simulink model "generic"  (R2022b)
settings: Solver=ode45  StartTime=0.0  StopTime=inf  RelTol=1e-3  EnableMultiTasking=on
values from neighbouring files (symbols this model uses):
  A = cell2mat(A_cell)    [MPCController1.m]    (also in MPC_Fmincon.m)
  B = cell2mat(B_cell)    [MPCController1.m]    (also in MPC_Fmincon.m)
  brake_select = ones(length(speed), length(steering_angle))    [TwoDLook_uptable.m]
  curvature = 0.000:0.001:1    [TwoDLook_uptable.m]
  m = 1600    [MPCController1.m]    (also in MPCController2.m; MPC_Fmincon.m)
  speed = 0:0.1:100    [TwoDLook_uptable.m]
undefined symbols (not defined in the file or in its folder): Amplifier, DiscIntNeverNeededParam, K_d_yawrate, K_dsteering, k_speed, k_stanley, kd, ki, kp, path_curvature
libraries: CarMaker4SL x97, simulink x6, cstblocks x6, simulink_extras x4, autolibshared x1, mpcadaslib x1
(part 4 of 6)

== system generic/CarMaker/VehicleControl/CreateBus VhclCtrl1/Stanley steering & speed//Brake controller/Stanley_controller_with_thottle_and_brake_commands/Stanley steering + PID speed controller/Smoothing ==
  Signal_In : Inport
  Add : Sum  Inputs=++++
  Delay : Delay  InitialCondition=0.1
  Delay1 : Delay  DelayLength=4  InitialCondition=0.1
  Delay2 : Delay  DelayLength=5  InitialCondition=0.1
  Gain : Gain  Gain=0.35
  Gain1 : Gain  Gain=0.25
  Gain2 : Gain  Gain=0.25
  Gain3 : Gain  Gain=0.15
  Signal_Out : Outport  VectorParamsAs1DForOutWhenUnconnected=off
  wires:
  Gain1/1 -> Add/2
  Signal_In/1 -> Gain/1
  Delay/1 -> Gain1/1
  Gain/1 -> Add/1
  Delay1/1 -> Gain2/1
  Add/1 -> Delay2/1, Delay1/1, Delay/1, Signal_Out/1
  Gain2/1 -> Add/3
  Delay2/1 -> Gain3/1
  Gain3/1 -> Add/4

== system generic/CarMaker/VehicleControl/CreateBus VhclCtrl1/Stanley steering & speed//Brake controller/Stanley_controller_with_thottle_and_brake_commands/Stanley steering + PID speed controller/Speed_controller ==
  path : Inport
  speed_act : Inport  Port=2
  velocity_x : Inport  Port=3
  velocity_y : Inport  Port=4
  desired_speed : Inport  Port=5
  steering : Inport  Port=6
  Brake Saturation : Saturate  UpperLimit=1  LowerLimit=0
  Constant1 : Constant  Value=kd
  Constant2 : Constant  Value=ki
  Constant3 : Constant  Value=kp
  Path_curvature : Constant  Value=path_curvature
  Scaling factor : Gain  Gain=1/1000
  Scalling factor : Gain  Gain=1/1000
  Throttle Saturation : Saturate  UpperLimit=1  LowerLimit=-1
  advancedPID_speed_and_brake_control : MATLAB Function  TreatAsAtomicUnit=on
  calculate_path_curvature : MATLAB Function  TreatAsAtomicUnit=on
  Throttle : Outport
  Brake_command : Outport  Port=2
  path_curvature : Outport  Port=3
  min_safe_speed : Outport  Port=4
  wires:
  advancedPID_speed_and_brake_control/1(throttle) -> Scaling factor/1  "throttle"
  path/1 -> calculate_path_curvature/1(path)
  speed_act/1 -> advancedPID_speed_and_brake_control/3(speed_act)
  calculate_path_curvature/2(min_safe_speed) -> min_safe_speed/1, advancedPID_speed_and_brake_control/2(min_s_speed)  "min_s_speed"
  velocity_y/1 -> calculate_path_curvature/2(velocity_y)
  velocity_x/1 -> calculate_path_curvature/3(velocity_x)
  steering/1 -> calculate_path_curvature/4(steering_angel)
  calculate_path_curvature/1(path_curvature) -> path_curvature/1
  Constant3/1 -> advancedPID_speed_and_brake_control/7(Kp_speed)
  Path_curvature/1 -> advancedPID_speed_and_brake_control/1(path_curv)
  desired_speed/1 -> advancedPID_speed_and_brake_control/4(desired_speed)
  Constant2/1 -> advancedPID_speed_and_brake_control/6(Ki_speed)
  Constant1/1 -> advancedPID_speed_and_brake_control/5(Kd_speed)
  advancedPID_speed_and_brake_control/2(brake_cmd) -> Scalling factor/1  "Brake cmd"
  Scaling factor/1 -> Throttle Saturation/1
  Throttle Saturation/1 -> Throttle/1  "Throttle_command"
  Scalling factor/1 -> Brake Saturation/1
  Brake Saturation/1 -> Brake_command/1  "Brake_command"

== system generic/CarMaker/VehicleControl/CreateBus VhclCtrl1/Stanley steering & speed//Brake controller/Stanley_controller_with_thottle_and_brake_commands/Stanley steering + PID speed controller/Subsystem1 ==
  desired_speed : Inport
  curvature : Inport  Port=2
  min_safe_speed : Inport  Port=3
  2-D Lookup Table : Lookup_n-D  BreakpointsForDimension1=speed  BreakpointsForDimension2=curvature  Table=brake_select  InternalRulePriority=Speed  RndMeth=Simplest
      settings: InputPortMap=u0,u1
  Divide : Product  Inputs=*/
  MATLAB Function : MATLAB Function  Commented=on  TreatAsAtomicUnit=on
  Read CM Dict : CarMaker4SL/Read CM Dict  xname=Sensor.Road.VehSensor_0.Path.CurveXY  xsync=off  xstime=Continuous
  Scope2 : Scope
  Target_speed : Outport
  curv : Outport  Port=2
  speed : Outport  Port=3
  wires:
  Divide/1 -> speed/1, Target_speed/1, Scope2/1
  2-D Lookup Table/1 -> Divide/2
  desired_speed/1 -> 2-D Lookup Table/1, Divide/1
  min_safe_speed/1 -> MATLAB Function/2(min_safe_speed)
  curvature/1 -> MATLAB Function/1(u)
  Read CM Dict/1 -> curv/1, 2-D Lookup Table/2

== system generic/CarMaker/VehicleControl/CreateBus VhclCtrl1/Stanley steering & speed//Brake controller/Road sensor set & path planning/Road sensor set & path planning/A* star path planning/Signal_smoothing ==
  Signal_In : Inport
  Smoothing1 : Subsystem
  Smoothing2 : Subsystem
  Smoothing4 : Subsystem
  smoothed_width : Outport
  wires:
  Signal_In/1 -> Smoothing1/1(Signal_In)
  Smoothing1/1(Signal_Out) -> Smoothing2/1(Signal_In)  "steering_signal"
  Smoothing2/1(Signal_Out) -> Smoothing4/1(Signal_In)  "steering_signal"
  Smoothing4/1(Signal_Out) -> smoothed_width/1  "smoothed_width"

== system generic/CarMaker/VehicleControl/CreateBus VhclCtrl1/Stanley steering & speed//Brake controller/Road sensor set & path planning/Road sensor set & path planning/A* star path planning/Smoothing3 ==
  Signal_In : Inport
  Add : Sum  Inputs=++++
  Delay : Delay  InitialCondition=0.1
  Delay1 : Delay  DelayLength=4  InitialCondition=0.1
  Delay2 : Delay  DelayLength=5  InitialCondition=0.1
  Gain : Gain  Gain=0.35
  Gain1 : Gain  Gain=0.25
  Gain2 : Gain  Gain=0.25
  Gain3 : Gain  Gain=0.15
  Signal_Out : Outport  VectorParamsAs1DForOutWhenUnconnected=off
  wires:
  Gain3/1 -> Add/4
  Delay2/1 -> Gain3/1
  Gain2/1 -> Add/3
  Add/1 -> Signal_Out/1, Delay/1, Delay1/1, Delay2/1
  Delay1/1 -> Gain2/1
  Gain/1 -> Add/1
  Delay/1 -> Gain1/1
  Signal_In/1 -> Gain/1
  Gain1/1 -> Add/2

== system generic/CarMaker/VehicleControl/CreateBus VhclCtrl1/Stanley steering & speed//Brake controller/Road sensor set & path planning/Road sensor set & path planning/Be'zeir path planning/Signal_smoothing ==
  Signal_In : Inport
  Smoothing1 : Subsystem
  Smoothing2 : Subsystem
  Smoothing4 : Subsystem
  smoothed_width : Outport
  wires:
  Smoothing4/1(Signal_Out) -> smoothed_width/1  "smoothed_width"
  Smoothing2/1(Signal_Out) -> Smoothing4/1(Signal_In)  "steering_signal"
  Smoothing1/1(Signal_Out) -> Smoothing2/1(Signal_In)  "steering_signal"
  Signal_In/1 -> Smoothing1/1(Signal_In)

== system generic/CarMaker/VehicleControl/CreateBus VhclCtrl1/Stanley steering & speed//Brake controller/Road sensor set & path planning/Road sensor set & path planning/Be'zeir path planning/Smoothing3 ==
  Signal_In : Inport
  Add : Sum  Inputs=++++
  Delay : Delay  InitialCondition=0.1
  Delay1 : Delay  DelayLength=4  InitialCondition=0.1
  Delay2 : Delay  DelayLength=5  InitialCondition=0.1
  Gain : Gain  Gain=0.35
  Gain1 : Gain  Gain=0.25
  Gain2 : Gain  Gain=0.25
  Gain3 : Gain  Gain=0.15
  Signal_Out : Outport  VectorParamsAs1DForOutWhenUnconnected=off
  wires:
  Gain1/1 -> Add/2
  Signal_In/1 -> Gain/1
  Delay/1 -> Gain1/1
  Gain/1 -> Add/1
  Delay1/1 -> Gain2/1
  Add/1 -> Delay2/1, Delay1/1, Delay/1, Signal_Out/1
  Gain2/1 -> Add/3
  Delay2/1 -> Gain3/1
  Gain3/1 -> Add/4

== system generic/CarMaker/VehicleControl/CreateBus VhclCtrl1/Stanley steering & speed//Brake controller/Road sensor set & path planning/Road sensor set & path planning/Car_yaw_rate/ Path_expanding1 ==
  X-path : Inport
  Y_path : Inport  Port=2
  Delay10 : Delay  DelayLength=6
  Delay11 : Delay  DelayLength=8
  Delay37 : Delay
  Delay38 : Delay  DelayLength=4
  Delay4 : Delay
  Delay5 : Delay  DelayLength=6
  Delay6 : Delay  DelayLength=8
  Delay9 : Delay  DelayLength=4
  Mux1 : Mux  Inputs=5
  Mux2 : Mux  Inputs=5
  Reshape1 : Reshape  OutputDimensionality=Customize  OutputDimensions=[1,5]
  Reshape2 : Reshape  OutputDimensionality=Customize  OutputDimensions=[1,5]
  x_path : Outport
  y_path : Outport  Port=2
  wires:
  Mux2/1 -> Reshape2/1
  Reshape2/1 -> x_path/1
  Delay11/1 -> Mux1/5
  Delay10/1 -> Mux1/4
  Delay9/1 -> Mux1/3
  Delay4/1 -> Mux1/2
  Reshape1/1 -> y_path/1
  Mux1/1 -> Reshape1/1
  Delay38/1 -> Mux2/3
  Delay6/1 -> Mux2/5
  Delay37/1 -> Mux2/2
  Delay5/1 -> Mux2/4
  Y_path/1 -> Delay11/1, Delay10/1, Delay9/1, Delay4/1, Mux1/1
  X-path/1 -> Delay6/1, Delay5/1, Delay37/1, Delay38/1, Mux2/1

== system generic/CarMaker/VehicleControl/CreateBus VhclCtrl1/Stanley steering & speed//Brake controller/Road sensor set & path planning/Road sensor set & path planning/Dijkestra path planning/Signal_smoothing ==
  Signal_In : Inport
  Smoothing1 : Subsystem
  Smoothing2 : Subsystem
  Smoothing4 : Subsystem
  smoothed_width : Outport
  wires:
  Smoothing4/1(Signal_Out) -> smoothed_width/1  "smoothed_width"
  Smoothing2/1(Signal_Out) -> Smoothing4/1(Signal_In)  "steering_signal"
  Smoothing1/1(Signal_Out) -> Smoothing2/1(Signal_In)  "steering_signal"
  Signal_In/1 -> Smoothing1/1(Signal_In)

== system generic/CarMaker/VehicleControl/CreateBus VhclCtrl1/Stanley steering & speed//Brake controller/Road sensor set & path planning/Road sensor set & path planning/Dijkestra path planning/Smoothing3 ==
  Signal_In : Inport
  Add : Sum  Inputs=++++
  Delay : Delay  InitialCondition=0.1
  Delay1 : Delay  DelayLength=4  InitialCondition=0.1
  Delay2 : Delay  DelayLength=5  InitialCondition=0.1
  Gain : Gain  Gain=0.35
  Gain1 : Gain  Gain=0.25
  Gain2 : Gain  Gain=0.25
  Gain3 : Gain  Gain=0.15
  Signal_Out : Outport  VectorParamsAs1DForOutWhenUnconnected=off
  wires:
  Gain1/1 -> Add/2
  Signal_In/1 -> Gain/1
  Delay/1 -> Gain1/1
  Gain/1 -> Add/1
  Delay1/1 -> Gain2/1
  Add/1 -> Delay2/1, Delay1/1, Delay/1, Signal_Out/1
  Gain2/1 -> Add/3
  Delay2/1 -> Gain3/1
  Gain3/1 -> Add/4

== system generic/CarMaker/VehicleControl/CreateBus VhclCtrl1/Stanley steering & speed//Brake controller/Road sensor set & path planning/Road sensor set & path planning/Path_curvature/ Path_expanding ==
  X-path : Inport
  Y_path : Inport  Port=2
  Delay10 : Delay  DelayLength=6
  Delay11 : Delay  DelayLength=8
  Delay37 : Delay
  Delay38 : Delay  DelayLength=4
  Delay4 : Delay
  Delay5 : Delay  DelayLength=6
  Delay6 : Delay  DelayLength=8
  Delay9 : Delay  DelayLength=4
  Mux1 : Mux  Inputs=5
  Mux2 : Mux  Inputs=5
  Reshape1 : Reshape  OutputDimensionality=Customize  OutputDimensions=[1,5]
  Reshape2 : Reshape  OutputDimensionality=Customize  OutputDimensions=[1,5]
  x_path : Outport
  y_path : Outport  Port=2
  wires:
  X-path/1 -> Mux2/1, Delay38/1, Delay37/1, Delay5/1, Delay6/1
  Y_path/1 -> Mux1/1, Delay4/1, Delay9/1, Delay10/1, Delay11/1
  Delay5/1 -> Mux2/4
  Delay37/1 -> Mux2/2
  Delay6/1 -> Mux2/5
  Delay38/1 -> Mux2/3
  Mux1/1 -> Reshape1/1
  Reshape1/1 -> y_path/1
  Delay4/1 -> Mux1/2
  Delay9/1 -> Mux1/3
  Delay10/1 -> Mux1/4
  Delay11/1 -> Mux1/5
  Reshape2/1 -> x_path/1
  Mux2/1 -> Reshape2/1

== system generic/CarMaker/VehicleControl/CreateBus VhclCtrl1/Stanley steering & speed//Brake controller/Road sensor set & path planning/Road sensor set & path planning/Spline_path_planning/Signal_smoothing ==
  Signal_In : Inport
  Smoothing1 : Subsystem
  Smoothing2 : Subsystem
  Smoothing4 : Subsystem
  smoothed_width : Outport
  wires:
  Signal_In/1 -> Smoothing1/1(Signal_In)
  Smoothing1/1(Signal_Out) -> Smoothing2/1(Signal_In)  "steering_signal"
  Smoothing2/1(Signal_Out) -> Smoothing4/1(Signal_In)  "steering_signal"
  Smoothing4/1(Signal_Out) -> smoothed_width/1  "smoothed_width"

== system generic/CarMaker/VehicleControl/CreateBus VhclCtrl1/Stanley steering & speed//Brake controller/Road sensor set & path planning/Road sensor set & path planning/Spline_path_planning/Smoothing3 ==
  Signal_In : Inport
  Add : Sum  Inputs=++++
  Delay : Delay  InitialCondition=0.1
  Delay1 : Delay  DelayLength=4  InitialCondition=0.1
  Delay2 : Delay  DelayLength=5  InitialCondition=0.1
  Gain : Gain  Gain=0.35
  Gain1 : Gain  Gain=0.25
  Gain2 : Gain  Gain=0.25
  Gain3 : Gain  Gain=0.15
  Signal_Out : Outport  VectorParamsAs1DForOutWhenUnconnected=off
  wires:
  Gain3/1 -> Add/4
  Delay2/1 -> Gain3/1
  Gain2/1 -> Add/3
  Add/1 -> Signal_Out/1, Delay/1, Delay1/1, Delay2/1
  Delay1/1 -> Gain2/1
  Gain/1 -> Add/1
  Delay/1 -> Gain1/1
  Signal_In/1 -> Gain/1
  Gain1/1 -> Add/2

== system generic/CarMaker/VehicleControl/CreateBus VhclCtrl1/Stanley steering & speed//Brake controller/Road sensor set & path planning/Road sensor set & path planning/path_planning/Signal_smoothing ==
  Signal_In : Inport
  Smoothing1 : Subsystem
  Smoothing2 : Subsystem
  Smoothing4 : Subsystem
  smoothed_width : Outport
  wires:
  Smoothing4/1(Signal_Out) -> smoothed_width/1  "smoothed_width"
  Smoothing2/1(Signal_Out) -> Smoothing4/1(Signal_In)  "steering_signal"
  Smoothing1/1(Signal_Out) -> Smoothing2/1(Signal_In)  "steering_signal"
  Signal_In/1 -> Smoothing1/1(Signal_In)

== system generic/CarMaker/VehicleControl/CreateBus VhclCtrl1/Stanley steering & speed//Brake controller/Road sensor set & path planning/Road sensor set & path planning/path_planning/Smoothing3 ==
  Signal_In : Inport
  Add : Sum  Inputs=++++
  Delay : Delay  InitialCondition=0.1
  Delay1 : Delay  DelayLength=4  InitialCondition=0.1
  Delay2 : Delay  DelayLength=5  InitialCondition=0.1
  Gain : Gain  Gain=0.35
  Gain1 : Gain  Gain=0.25
  Gain2 : Gain  Gain=0.25
  Gain3 : Gain  Gain=0.15
  Signal_Out : Outport  VectorParamsAs1DForOutWhenUnconnected=off
  wires:
  Gain1/1 -> Add/2
  Signal_In/1 -> Gain/1
  Delay/1 -> Gain1/1
  Gain/1 -> Add/1
  Delay1/1 -> Gain2/1
  Add/1 -> Delay2/1, Delay1/1, Delay/1, Signal_Out/1
  Gain2/1 -> Add/3
  Delay2/1 -> Gain3/1
  Gain3/1 -> Add/4

== system generic/CarMaker/VehicleControl/CreateBus VhclCtrl1/Stanley steering & speed//Brake controller/Stanley_controller_vfin/Stanley_controller_vfin/Stanley_standfort controller/Crosstrack_steering ==
  speed : Inport
  Path.DevDist : Inport  Port=2
  Atan : Trigonometry  Operator=atan
  Divide : Product  Inputs=*/
  Gain : Gain  Gain=-1
  Product : Product
  Sum1 : Sum  Inputs=|++
  k_speed : Constant  Value=k_speed
  k_stanley : Constant  Value=k_stanley
  Cross_track_steering : Outport
  wires:
  Atan/1 -> Cross_track_steering/1
  Divide/1 -> Atan/1
  k_speed/1 -> Sum1/1
  speed/1 -> Sum1/2
  k_stanley/1 -> Product/2
  Sum1/1 -> Divide/2
  Product/1 -> Gain/1
  Gain/1 -> Divide/1
  Path.DevDist/1 -> Product/1

== system generic/CarMaker/VehicleControl/CreateBus VhclCtrl1/Stanley steering & speed//Brake controller/Stanley_controller_vfin/Stanley_controller_vfin/Stanley_standfort controller/Deviation_angle_calc ==
  Velocity : Inport
  Curvature : Inport  Port=2
  Car.YawRate : Inport  Port=3
  Amplifyer : Gain  Gain=Amplifier
  Amplifyer1 : Gain  Gain=10
  Amplifyer2 : Gain  Gain=16.56
  Constant : Constant  Value=2
  Discrete-Time Integrator : DiscreteIntegrator  SampleTime=-1  ICPrevOutput=DiscIntNeverNeededParam  ICPrevScaledInput=DiscIntNeverNeededParam
  Integrator : DiscreteIntegrator  SampleTime=-1  ICPrevOutput=DiscIntNeverNeededParam  ICPrevScaledInput=DiscIntNeverNeededParam
  Multiport Switch : MultiPortSwitch  Inputs=2  SaturateOnIntegerOverflow=off  InputSameDT=off
  Product : Product
  Read CM Dict : CarMaker4SL/Read CM Dict  xname=Sensor.Road.VehSensor_0.Path.DevAng  xsync=off  xstime=Continuous
  Scope : Scope  NumInputPorts=2
  Sum3 : Sum  Inputs=|+-
  Switch : Switch  Criteria=u2 > Threshold  SaturateOnIntegerOverflow=off  InputSameDT=off
  Dev_angle : Outport
  wires:
  Amplifyer1/1 -> Switch/3  "Dev_angle"
  Curvature/1 -> Product/1
  Car.YawRate/1 -> Discrete-Time Integrator/1
  Velocity/1 -> Product/2
  Product/1 -> Integrator/1
  Integrator/1 -> Sum3/1  "Dev_angle"
  Discrete-Time Integrator/1 -> Sum3/2
  Amplifyer2/1 -> Switch/1  "Dev_angle"
  Sum3/1 -> Amplifyer1/1, Switch/2, Amplifyer2/1  "heading_error"
  Switch/1 -> Scope/1, Multiport Switch/2  "Dev_angle"
  Amplifyer/1 -> Scope/2, Multiport Switch/3  "Dev_angle"
  Read CM Dict/1 -> Amplifyer/1
  Constant/1 -> Multiport Switch/1
  Multiport Switch/1 -> Dev_angle/1  "Dev_angle"

== system generic/CarMaker/VehicleControl/CreateBus VhclCtrl1/Stanley steering & speed//Brake controller/Stanley_controller_vfin/Stanley_controller_vfin/Stanley_standfort controller/Steady_state_yaw ==
  V : Inport
  Curvature : Inport  Port=2
  Car_Yaw_rate : Inport  Port=3
  Discrete-Time Integrator : DiscreteIntegrator  SampleTime=-1  ICPrevOutput=DiscIntNeverNeededParam  ICPrevScaledInput=DiscIntNeverNeededParam
  Steady_state_yaw : Subsystem
  Sum : Sum  Inputs=|-+
  Steady_state_yaw1 : Outport
  wires:
  V/1 -> Steady_state_yaw/1(V)
  Sum/1 -> Steady_state_yaw1/1  "Steady_state_yaw"
  Steady_state_yaw/1(Steady_state_yaw) -> Sum/1  "Steady_state_yaw"
  Discrete-Time Integrator/1 -> Sum/2
  Car_Yaw_rate/1 -> Discrete-Time Integrator/1
  Curvature/1 -> Steady_state_yaw/2(Curvature)

== system generic/CarMaker/VehicleControl/CreateBus VhclCtrl1/Stanley steering & speed//Brake controller/Stanley_controller_vfin/Stanley_controller_vfin/Stanley_standfort controller/Steering_correction_facotr ==
  Steering_i+1 : Inport
  Steering_i : Inport  Port=2
  K_dsteering : Constant  Value=K_dsteering
  Memory : Memory  LinearizeAsDelay=on
  Product2 : Product
  Sum2 : Sum  Inputs=|+-
  Factor_of_correction : Outport
  wires:
  K_dsteering/1 -> Product2/1
  Memory/1 -> Sum2/1
  Sum2/1 -> Product2/2
  Steering_i+1/1 -> Sum2/2
  Steering_i/1 -> Memory/1
  Product2/1 -> Factor_of_correction/1

== system generic/CarMaker/VehicleControl/CreateBus VhclCtrl1/Stanley steering & speed//Brake controller/Stanley_controller_vfin/Stanley_controller_vfin/Stanley_standfort controller/Yaw_rate_diff ==
  Velocity : Inport
  Curvature : Inport  Port=2
  Car_yaw_rate : Inport  Port=3
  K_d_yawrate : Constant  Value=K_d_yawrate
  Product : Product
  Product1 : Product
  Sum1 : Sum  Inputs=|+-
  Yaw_rate_factor : Outport
  wires:
  K_d_yawrate/1 -> Product1/1
  Car_yaw_rate/1 -> Sum1/2
  Velocity/1 -> Product/1
  Curvature/1 -> Product/2
  Sum1/1 -> Product1/2
  Product/1 -> Sum1/1
  Product1/1 -> Yaw_rate_factor/1

== system generic/CarMaker/VehicleControl/CreateBus VhclCtrl1/Stanley steering & speed//Brake controller/Road sensor set & path planning/Road sensor set & path planning/A* star path planning/Signal_smoothing/Smoothing1 ==
  Signal_In : Inport
  Add : Sum  Inputs=++++
  Delay : Delay  InitialCondition=0.1
  Delay1 : Delay  DelayLength=4  InitialCondition=0.1
  Delay2 : Delay  DelayLength=5  InitialCondition=0.1
  Gain : Gain  Gain=0.35
  Gain1 : Gain  Gain=0.25
  Gain2 : Gain  Gain=0.25
  Gain3 : Gain  Gain=0.15
  Signal_Out : Outport  VectorParamsAs1DForOutWhenUnconnected=off
  wires:
  Gain1/1 -> Add/2
  Signal_In/1 -> Gain/1
  Delay/1 -> Gain1/1
  Gain/1 -> Add/1
  Delay1/1 -> Gain2/1
  Add/1 -> Delay2/1, Delay1/1, Delay/1, Signal_Out/1
  Gain2/1 -> Add/3
  Delay2/1 -> Gain3/1
  Gain3/1 -> Add/4

== system generic/CarMaker/VehicleControl/CreateBus VhclCtrl1/Stanley steering & speed//Brake controller/Road sensor set & path planning/Road sensor set & path planning/A* star path planning/Signal_smoothing/Smoothing2 ==
  Signal_In : Inport
  Add : Sum  Inputs=++++
  Delay : Delay  InitialCondition=0.1
  Delay1 : Delay  DelayLength=4  InitialCondition=0.1
  Delay2 : Delay  DelayLength=5  InitialCondition=0.1
  Gain : Gain  Gain=0.35
  Gain1 : Gain  Gain=0.25
  Gain2 : Gain  Gain=0.25
  Gain3 : Gain  Gain=0.15
  Signal_Out : Outport  VectorParamsAs1DForOutWhenUnconnected=off
  wires:
  Gain3/1 -> Add/4
  Delay2/1 -> Gain3/1
  Gain2/1 -> Add/3
  Add/1 -> Signal_Out/1, Delay/1, Delay1/1, Delay2/1
  Delay1/1 -> Gain2/1
  Gain/1 -> Add/1
  Delay/1 -> Gain1/1
  Signal_In/1 -> Gain/1
  Gain1/1 -> Add/2

== system generic/CarMaker/VehicleControl/CreateBus VhclCtrl1/Stanley steering & speed//Brake controller/Road sensor set & path planning/Road sensor set & path planning/A* star path planning/Signal_smoothing/Smoothing4 ==
  Signal_In : Inport
  Add : Sum  Inputs=++++
  Delay : Delay  InitialCondition=0.1
  Delay1 : Delay  DelayLength=4  InitialCondition=0.1
  Delay2 : Delay  DelayLength=5  InitialCondition=0.1
  Gain : Gain  Gain=0.35
  Gain1 : Gain  Gain=0.25
  Gain2 : Gain  Gain=0.25
  Gain3 : Gain  Gain=0.15
  Signal_Out : Outport  VectorParamsAs1DForOutWhenUnconnected=off
  wires:
  Gain1/1 -> Add/2
  Signal_In/1 -> Gain/1
  Delay/1 -> Gain1/1
  Gain/1 -> Add/1
  Delay1/1 -> Gain2/1
  Add/1 -> Delay2/1, Delay1/1, Delay/1, Signal_Out/1
  Gain2/1 -> Add/3
  Delay2/1 -> Gain3/1
  Gain3/1 -> Add/4

== system generic/CarMaker/VehicleControl/CreateBus VhclCtrl1/Stanley steering & speed//Brake controller/Road sensor set & path planning/Road sensor set & path planning/Be'zeir path planning/Signal_smoothing/Smoothing1 ==
  Signal_In : Inport
  Add : Sum  Inputs=++++
  Delay : Delay  InitialCondition=0.1
  Delay1 : Delay  DelayLength=4  InitialCondition=0.1
  Delay2 : Delay  DelayLength=5  InitialCondition=0.1
  Gain : Gain  Gain=0.35
  Gain1 : Gain  Gain=0.25
  Gain2 : Gain  Gain=0.25
  Gain3 : Gain  Gain=0.15
  Signal_Out : Outport  VectorParamsAs1DForOutWhenUnconnected=off
  wires:
  Gain3/1 -> Add/4
  Delay2/1 -> Gain3/1
  Gain2/1 -> Add/3
  Add/1 -> Signal_Out/1, Delay/1, Delay1/1, Delay2/1
  Delay1/1 -> Gain2/1
  Gain/1 -> Add/1
  Delay/1 -> Gain1/1
  Signal_In/1 -> Gain/1
  Gain1/1 -> Add/2

== system generic/CarMaker/VehicleControl/CreateBus VhclCtrl1/Stanley steering & speed//Brake controller/Road sensor set & path planning/Road sensor set & path planning/Be'zeir path planning/Signal_smoothing/Smoothing2 ==
  Signal_In : Inport
  Add : Sum  Inputs=++++
  Delay : Delay  InitialCondition=0.1
  Delay1 : Delay  DelayLength=4  InitialCondition=0.1
  Delay2 : Delay  DelayLength=5  InitialCondition=0.1
  Gain : Gain  Gain=0.35
  Gain1 : Gain  Gain=0.25
  Gain2 : Gain  Gain=0.25
  Gain3 : Gain  Gain=0.15
  Signal_Out : Outport  VectorParamsAs1DForOutWhenUnconnected=off
  wires:
  Gain1/1 -> Add/2
  Signal_In/1 -> Gain/1
  Delay/1 -> Gain1/1
  Gain/1 -> Add/1
  Delay1/1 -> Gain2/1
  Add/1 -> Delay2/1, Delay1/1, Delay/1, Signal_Out/1
  Gain2/1 -> Add/3
  Delay2/1 -> Gain3/1
  Gain3/1 -> Add/4

== system generic/CarMaker/VehicleControl/CreateBus VhclCtrl1/Stanley steering & speed//Brake controller/Road sensor set & path planning/Road sensor set & path planning/Be'zeir path planning/Signal_smoothing/Smoothing4 ==
  Signal_In : Inport
  Add : Sum  Inputs=++++
  Delay : Delay  InitialCondition=0.1
  Delay1 : Delay  DelayLength=4  InitialCondition=0.1
  Delay2 : Delay  DelayLength=5  InitialCondition=0.1
  Gain : Gain  Gain=0.35
  Gain1 : Gain  Gain=0.25
  Gain2 : Gain  Gain=0.25
  Gain3 : Gain  Gain=0.15
  Signal_Out : Outport  VectorParamsAs1DForOutWhenUnconnected=off
  wires:
  Gain3/1 -> Add/4
  Delay2/1 -> Gain3/1
  Gain2/1 -> Add/3
  Add/1 -> Signal_Out/1, Delay/1, Delay1/1, Delay2/1
  Delay1/1 -> Gain2/1
  Gain/1 -> Add/1
  Delay/1 -> Gain1/1
  Signal_In/1 -> Gain/1
  Gain1/1 -> Add/2

== system generic/CarMaker/VehicleControl/CreateBus VhclCtrl1/Stanley steering & speed//Brake controller/Road sensor set & path planning/Road sensor set & path planning/Dijkestra path planning/Signal_smoothing/Smoothing1 ==
  Signal_In : Inport
  Add : Sum  Inputs=++++
  Delay : Delay  InitialCondition=0.1
  Delay1 : Delay  DelayLength=4  InitialCondition=0.1
  Delay2 : Delay  DelayLength=5  InitialCondition=0.1
  Gain : Gain  Gain=0.35
  Gain1 : Gain  Gain=0.25
  Gain2 : Gain  Gain=0.25
  Gain3 : Gain  Gain=0.15
  Signal_Out : Outport  VectorParamsAs1DForOutWhenUnconnected=off
  wires:
  Gain3/1 -> Add/4
  Delay2/1 -> Gain3/1
  Gain2/1 -> Add/3
  Add/1 -> Signal_Out/1, Delay/1, Delay1/1, Delay2/1
  Delay1/1 -> Gain2/1
  Gain/1 -> Add/1
  Delay/1 -> Gain1/1
  Signal_In/1 -> Gain/1
  Gain1/1 -> Add/2

== system generic/CarMaker/VehicleControl/CreateBus VhclCtrl1/Stanley steering & speed//Brake controller/Road sensor set & path planning/Road sensor set & path planning/Dijkestra path planning/Signal_smoothing/Smoothing2 ==
  Signal_In : Inport
  Add : Sum  Inputs=++++
  Delay : Delay  InitialCondition=0.1
  Delay1 : Delay  DelayLength=4  InitialCondition=0.1
  Delay2 : Delay  DelayLength=5  InitialCondition=0.1
  Gain : Gain  Gain=0.35
  Gain1 : Gain  Gain=0.25
  Gain2 : Gain  Gain=0.25
  Gain3 : Gain  Gain=0.15
  Signal_Out : Outport  VectorParamsAs1DForOutWhenUnconnected=off
  wires:
  Gain1/1 -> Add/2
  Signal_In/1 -> Gain/1
  Delay/1 -> Gain1/1
  Gain/1 -> Add/1
  Delay1/1 -> Gain2/1
  Add/1 -> Delay2/1, Delay1/1, Delay/1, Signal_Out/1
  Gain2/1 -> Add/3
  Delay2/1 -> Gain3/1
  Gain3/1 -> Add/4

== system generic/CarMaker/VehicleControl/CreateBus VhclCtrl1/Stanley steering & speed//Brake controller/Road sensor set & path planning/Road sensor set & path planning/Dijkestra path planning/Signal_smoothing/Smoothing4 ==
  Signal_In : Inport
  Add : Sum  Inputs=++++
  Delay : Delay  InitialCondition=0.1
  Delay1 : Delay  DelayLength=4  InitialCondition=0.1
  Delay2 : Delay  DelayLength=5  InitialCondition=0.1
  Gain : Gain  Gain=0.35
  Gain1 : Gain  Gain=0.25
  Gain2 : Gain  Gain=0.25
  Gain3 : Gain  Gain=0.15
  Signal_Out : Outport  VectorParamsAs1DForOutWhenUnconnected=off
  wires:
  Gain3/1 -> Add/4
  Delay2/1 -> Gain3/1
  Gain2/1 -> Add/3
  Add/1 -> Signal_Out/1, Delay/1, Delay1/1, Delay2/1
  Delay1/1 -> Gain2/1
  Gain/1 -> Add/1
  Delay/1 -> Gain1/1
  Signal_In/1 -> Gain/1
  Gain1/1 -> Add/2

== system generic/CarMaker/VehicleControl/CreateBus VhclCtrl1/Stanley steering & speed//Brake controller/Road sensor set & path planning/Road sensor set & path planning/Spline_path_planning/Signal_smoothing/Smoothing1 ==
  Signal_In : Inport
  Add : Sum  Inputs=++++
  Delay : Delay  InitialCondition=0.1
  Delay1 : Delay  DelayLength=4  InitialCondition=0.1
  Delay2 : Delay  DelayLength=5  InitialCondition=0.1
  Gain : Gain  Gain=0.35
  Gain1 : Gain  Gain=0.25
  Gain2 : Gain  Gain=0.25
  Gain3 : Gain  Gain=0.15
  Signal_Out : Outport  VectorParamsAs1DForOutWhenUnconnected=off
  wires:
  Gain1/1 -> Add/2
  Signal_In/1 -> Gain/1
  Delay/1 -> Gain1/1
  Gain/1 -> Add/1
  Delay1/1 -> Gain2/1
  Add/1 -> Delay2/1, Delay1/1, Delay/1, Signal_Out/1
  Gain2/1 -> Add/3
  Delay2/1 -> Gain3/1
  Gain3/1 -> Add/4

== system generic/CarMaker/VehicleControl/CreateBus VhclCtrl1/Stanley steering & speed//Brake controller/Road sensor set & path planning/Road sensor set & path planning/Spline_path_planning/Signal_smoothing/Smoothing2 ==
  Signal_In : Inport
  Add : Sum  Inputs=++++
  Delay : Delay  InitialCondition=0.1
  Delay1 : Delay  DelayLength=4  InitialCondition=0.1
  Delay2 : Delay  DelayLength=5  InitialCondition=0.1
  Gain : Gain  Gain=0.35
  Gain1 : Gain  Gain=0.25
  Gain2 : Gain  Gain=0.25
  Gain3 : Gain  Gain=0.15
  Signal_Out : Outport  VectorParamsAs1DForOutWhenUnconnected=off
  wires:
  Gain3/1 -> Add/4
  Delay2/1 -> Gain3/1
  Gain2/1 -> Add/3
  Add/1 -> Signal_Out/1, Delay/1, Delay1/1, Delay2/1
  Delay1/1 -> Gain2/1
  Gain/1 -> Add/1
  Delay/1 -> Gain1/1
  Signal_In/1 -> Gain/1
  Gain1/1 -> Add/2

== system generic/CarMaker/VehicleControl/CreateBus VhclCtrl1/Stanley steering & speed//Brake controller/Road sensor set & path planning/Road sensor set & path planning/Spline_path_planning/Signal_smoothing/Smoothing4 ==
  Signal_In : Inport
  Add : Sum  Inputs=++++
  Delay : Delay  InitialCondition=0.1
  Delay1 : Delay  DelayLength=4  InitialCondition=0.1
  Delay2 : Delay  DelayLength=5  InitialCondition=0.1
  Gain : Gain  Gain=0.35
  Gain1 : Gain  Gain=0.25
  Gain2 : Gain  Gain=0.25
  Gain3 : Gain  Gain=0.15
  Signal_Out : Outport  VectorParamsAs1DForOutWhenUnconnected=off
  wires:
  Gain1/1 -> Add/2
  Signal_In/1 -> Gain/1
  Delay/1 -> Gain1/1
  Gain/1 -> Add/1
  Delay1/1 -> Gain2/1
  Add/1 -> Delay2/1, Delay1/1, Delay/1, Signal_Out/1
  Gain2/1 -> Add/3
  Delay2/1 -> Gain3/1
  Gain3/1 -> Add/4

== system generic/CarMaker/VehicleControl/CreateBus VhclCtrl1/Stanley steering & speed//Brake controller/Road sensor set & path planning/Road sensor set & path planning/path_planning/Signal_smoothing/Smoothing1 ==
  Signal_In : Inport
  Add : Sum  Inputs=++++
  Delay : Delay  InitialCondition=0.1
  Delay1 : Delay  DelayLength=4  InitialCondition=0.1
  Delay2 : Delay  DelayLength=5  InitialCondition=0.1
  Gain : Gain  Gain=0.35
  Gain1 : Gain  Gain=0.25
  Gain2 : Gain  Gain=0.25
  Gain3 : Gain  Gain=0.15
  Signal_Out : Outport  VectorParamsAs1DForOutWhenUnconnected=off
  wires:
  Gain3/1 -> Add/4
  Delay2/1 -> Gain3/1
  Gain2/1 -> Add/3
  Add/1 -> Signal_Out/1, Delay/1, Delay1/1, Delay2/1
  Delay1/1 -> Gain2/1
  Gain/1 -> Add/1
  Delay/1 -> Gain1/1
  Signal_In/1 -> Gain/1
  Gain1/1 -> Add/2

== system generic/CarMaker/VehicleControl/CreateBus VhclCtrl1/Stanley steering & speed//Brake controller/Road sensor set & path planning/Road sensor set & path planning/path_planning/Signal_smoothing/Smoothing2 ==
  Signal_In : Inport
  Add : Sum  Inputs=++++
  Delay : Delay  InitialCondition=0.1
  Delay1 : Delay  DelayLength=4  InitialCondition=0.1
  Delay2 : Delay  DelayLength=5  InitialCondition=0.1
  Gain : Gain  Gain=0.35
  Gain1 : Gain  Gain=0.25
  Gain2 : Gain  Gain=0.25
  Gain3 : Gain  Gain=0.15
  Signal_Out : Outport  VectorParamsAs1DForOutWhenUnconnected=off
  wires:
  Gain1/1 -> Add/2
  Signal_In/1 -> Gain/1
  Delay/1 -> Gain1/1
  Gain/1 -> Add/1
  Delay1/1 -> Gain2/1
  Add/1 -> Delay2/1, Delay1/1, Delay/1, Signal_Out/1
  Gain2/1 -> Add/3
  Delay2/1 -> Gain3/1
  Gain3/1 -> Add/4

== system generic/CarMaker/VehicleControl/CreateBus VhclCtrl1/Stanley steering & speed//Brake controller/Road sensor set & path planning/Road sensor set & path planning/path_planning/Signal_smoothing/Smoothing4 ==
  Signal_In : Inport
  Add : Sum  Inputs=++++
  Delay : Delay  InitialCondition=0.1
  Delay1 : Delay  DelayLength=4  InitialCondition=0.1
  Delay2 : Delay  DelayLength=5  InitialCondition=0.1
  Gain : Gain  Gain=0.35
  Gain1 : Gain  Gain=0.25
  Gain2 : Gain  Gain=0.25
  Gain3 : Gain  Gain=0.15
  Signal_Out : Outport  VectorParamsAs1DForOutWhenUnconnected=off
  wires:
  Gain3/1 -> Add/4
  Delay2/1 -> Gain3/1
  Gain2/1 -> Add/3
  Add/1 -> Signal_Out/1, Delay/1, Delay1/1, Delay2/1
  Delay1/1 -> Gain2/1
  Gain/1 -> Add/1
  Delay/1 -> Gain1/1
  Signal_In/1 -> Gain/1
  Gain1/1 -> Add/2

== system generic/CarMaker/VehicleControl/CreateBus VhclCtrl1/Stanley steering & speed//Brake controller/Stanley_controller_vfin/Stanley_controller_vfin/Stanley_standfort controller/Steady_state_yaw/Steady_state_yaw ==
  V : Inport
  Curvature : Inport  Port=2
  Constant : Constant  Value=1600.004
  Constant1 : Constant  Value=70551.0
  Constant3 : Constant  Value=1.488
  Constant4 : Constant  Value=1.487
  Constant5 : Constant
  Divide : Product  Inputs=*/
  Divide1 : Product  Inputs=*/
  Gain : Gain  Gain=180/pi()
  Product : Product  Inputs=3
  Product1 : Product
  Square : Math  Operator=square
  Sum : Sum  Inputs=|++
  Steady_state_yaw : Outport
  wires:
  Square/1 -> Product/1
  Constant4/1 -> Divide/1
  Constant5/1 -> Sum/1
  Constant3/1 -> Divide/2
  V/1 -> Square/1
  Divide/1 -> Sum/2
  Sum/1 -> Product1/2
  Constant/1 -> Product/2
  Curvature/1 -> Product/3
  Constant1/1 -> Gain/1
  Product/1 -> Divide1/1
  Product1/1 -> Divide1/2
  Divide1/1 -> Steady_state_yaw/1
  Gain/1 -> Product1/1

== matlab function generic/CarMaker/VehicleControl/CreateBus VhclCtrl1/MPC_steering_controllers/Subsystem/MATLAB Function5 ==
  data: x input; u input; u_optimal output; dt input; delta output; v_longitudinal output; path_ref input
function [u_optimal, delta, v_longitudinal] = MPCControllerPathTrackingWithHeadingError(x, u, dt,path_ref)
    function lateral_deviation = calculateLateralDeviation(x, path_ref)
        % Calculate lateral deviation from the reference path
        x_ref = path_ref(1, :);
        y_ref = path_ref(2, :);
    
        x_car = x(3);  % Lateral position of the car
        y_car = x(4);  % Yaw angle of the car
    
        % Rotate the car's coordinates to the reference path frame
        x_car_rot = cos(-x(4)) * (x_car - x_ref) - sin(-x(4)) * (y_car - y_ref);
        y_car_rot = sin(-x(4)) * (x_car - x_ref) + cos(-x(4)) * (y_car - y_ref);
    
        % Calculate lateral deviation
        lateral_deviation = y_car_rot;
    end
    % Adaptive Model Predictive Controller (Adaptive MPC) for steering control
    % Define system parameters (replace these with your actual vehicle parameters)
    lf = 1.449;  % Distance from centre of gravity to the front axle [m]
    m = 1600.0; % Kg
    lr = 1.449;   % Distance from centre of gravity to the Rear axle  [m]
    I = m*(lf+lr)^2/12;   % Carbody.inertia.z [Kgm2], assuming a rectangular shape
    theta = [0.1; 0.1];
    alpha = 0.1;
    cr = 160000; % Slip stiffness rear axle [N/rad]
    cf = 100000; % Slip stiffness Front axle [N/rad]
    % Define MPC parameters (modify as needed)
    N = 5;  % Prediction horizon
    Q = diag([1, 1, 10, 1, 1]);  % State cost matrix (including heading error)
    R = diag([0.1, 0.1]);  % Input cost matrix

    % Define state-space model
    A = [-2 * (cf + cr) / (m * u(2)), -u(2) - 2 * (cf * lf - cr * lr) / (m * u(2)); ...
         -2 * (cf * lf - cr * lr) / (m * u(2)), -2 * (cf * lf^2 + cr * lr^2) / (m * u(2))];
    B = [2 * cf / m, 0; 2 * cf * lf / (m * u(2)), 0];

    % Construct matrices for quadratic programming
    Qbar = blkdiag(kron(eye(N), Q), eye(N));  % State cost matrix for prediction horizon
    Rbar = kron(eye(N), R);  % Input cost matrix for prediction horizon
    
    % Ensure Qbar has the correct size
    Qbar = reshape(Qbar, [size(Qbar, 1), size(Qbar, 2)]);
    
    % Ensure x has the correct size
    x = reshape(x, [numel(x), 1]);
    
    % Initialize the Hessian matrix
    H = zeros(size(B, 2), size(B, 2));
    disp(Q)
    % Perform element-wise multiplication for each block in Qbar
    for i = 1:N
        H = H + B' * Qbar((i-1)*size(Q, 1) + 1:i*size(Q, 1), (i-1)*size(Q, 2) + 1:i*size(Q, 2)) * B;
    end

    % Add the Rbar term
    H = H + Rbar(1:2, 1:2);
    
    % Ensure x has the correct size for element-wise multiplication
    x = reshape(x, [numel(x), 1]);
    
    % Initialize the linear term
    f = zeros(size(B, 2), 1);
    
    % Perform element-wise multiplication for each block in Qbar
    for i = 1:N
        f = f + B' * Qbar((i-1)*size(Q, 1) + 1:i*size(Q, 1), (i-1)*size(Q, 2) + 1:i*size(Q, 2)) * x;
    end
    
    % Ensure f has the correct size
    f = reshape(f, [numel(f), 1]);


    % Define inequality constraints for longitudinal velocity
    Aineq = [0, 1; 0, -1];
    Bineq = [5 - u(2); u(2) - 5];

    % Solve quadratic programming problem
    options = optimoptions('fmincon', 'Display', 'off', 'Algorithm', 'sqp');
    % Initialize delta_u
    u0 = zeros(size(B, 2), 1);
    
    % Solve quadratic programming problem using fmincon
    delta_u = fmincon(@(u) 0.5 * u' * H * u + f' * u, u0, Aineq, Bineq, [], [], [], [], [], options);
    
    % Extract the optimal input from the solution
    u_optimal = delta_u(1:2);



    % Initialize x_new
    x_new = x;
    
    % Update state using the model
    x_new(1:2) = x_new(1:2) + (A(1:2, 1:2) * x(1:2) + B(1:2, :) * u_optimal) * dt;
    x_new(3:4) = x_new(3:4) + (A(3:4, 3:4) * x_new(3:4) + B(3:4, :) * u_optimal) * dt;
    
    % Initialize x_next
    x_next = zeros(size(x_new));
    
    % Adaptive parameter update (gradient descent)
    x_next(1:2) = x_new(1:2) + (A(1:2, 1:2) * x_new(1:2) + B(1:2, :) * u_optimal) * dt;
    x_next(3:4) = x_next(3:4) + (A(3:4, 3:4) * x_next(3:4) + B(3:4, :) * u_optimal) * dt;
    
    theta_new = theta - alpha * ((x_next(1:2) - x_new(1:2)) * x(1:2)');



    % Calculate lateral deviation from the reference path
    lateral_deviation = calculateLateralDeviation(x_new, path_ref);

    % Calculate heading error
    heading_error = x_new(4) - atan2(path_ref(2, end) - path_ref(2, 1), path_ref(1, end) - path_ref(1, 1));

    % Cost function modification for path tracking with heading error
    cost = lateral_deviation' * Q(3,3) * lateral_deviation + heading_error^2 + delta_u' * R * delta_u;

    % Extract control input (steering angle and longitudinal velocity) from the optimization result
    delta = u_optimal(1);
    v_longitudinal = u_optimal(2);

end

== matlab function generic/CarMaker/VehicleControl/CreateBus VhclCtrl1/Stanley steering & speed//Brake controller/Stanley_controller_with_thottle_and_brake_commands/Stanley steering + PID speed controller/Subsystem1/MATLAB Function ==
  data: u input; curv output; min_safe_speed input; speed output
function [curv, speed] = fcn(u, min_safe_speed)

curv = abs(max(u));
speed = max(min_safe_speed);

== matlab function generic/CarMaker/VehicleControl/CreateBus VhclCtrl1/MPC_steering_controllers/Subsystem/MATLAB Function3 ==
  data: x input; u input; u_optimal output; dt input; x_new output; theta_new output
function [u_optimal, x_new,theta_new] = adaptive_steering_mpc(x,u,dt)
    % Adaptive Model Predictive Controller (Adaptive MPC) for steering control
    % Define system parameters (replace these with your actual vehicle parameters)
    lf = 1.449;  % Distance from centre of gravity to the front axle [m]
    lr = 1.449;   % Distance from centre of gravity to the Rear axle  [m]
    I = m*(lf+lr)^2/12;   % Carbody.inertia.z [Kgm2], assuming a rectangular shape
    
    cr = 160000; % Slip stiffness rear axle [N/rad]
    cf = 100000; % Slip stiffness Front axle [N/rad]
    % Define MPC parameters (modify as needed)
    N = 5;  % Prediction horizon
    Q = eye(4);  % State cost matrix
    R = eye(2);  % Input cost matrix

    % Define state-space model
    A = [-2 * (cf + cr) / (m * u(2)), -u(2) - 2 * (cf * lf - cr * lr) / (m * u(2)); ...
         -2 * (cf * lf - cr * lr) / (m * u(2)), -2 * (cf * lf^2 + cr * lr^2) / (m * u(2))];
    B = [2 * cf / m, 0; 2 * cf * lf / (m * u(2)), 0];

    % Construct matrices for quadratic programming
    Qbar = blkdiag(kron(eye(N), Q), eye(N));  % State cost matrix for prediction horizon
    Rbar = kron(eye(N), R);  % Input cost matrix for prediction horizon
    H = B' * Qbar * B + Rbar;  % Hessian matrix
    f = (x' * Qbar * B)';  % Linear term

    % Solve quadratic programming problem
    options = optimset('Display', 'off');
    delta_u = quadprog(H, f, [], [], [], [], [], [], [], options);

    % Extract the optimal input from the solution
    u_optimal = delta_u(1:2);

    % Update state using the model
    x_new = x + (A * x + B * u_optimal) * dt;

    % Adaptive parameter update (gradient descent)
    x_next = x_new + (A * x_new + B * u_optimal) * dt;
    theta_new = theta - alpha * (x_next - x_new) * x';
end

== matlab function generic/CarMaker/VehicleControl/CreateBus VhclCtrl1/MPC_steering_controllers/Subsystem/MATLAB Function4 ==
  data: heading_error input; delta output; u2 input
function delta = ampc_steering_control(heading_error, u2)
    persistent model_params
    function params = initialize_model_params()
        % Define the vehicle parameters
        m = 2100;  % Car body mass [Kg]
        lf = 1.2;  % Distance from center of gravity to the front axle [m]
        lr = 1.6;  % Distance from center of gravity to the rear axle [m]
        I = m * (lf + lr)^2 / 12;  % Car body inertia [Kgm^2]
    
        cr = 160000;  % Slip stiffness rear axle [N/rad]
        cf = 100000;  % Slip stiffness front axle [N/rad]
    
        % Define the state-space model
        A = [-2 * (cf + cr) / m, -u2; -2 * (cf * lf - cr * lr) / I, -2 * (cf * lf^2 + cr * lr^2) / I];
        B = [2 * cf / m; 2 * cf * lf / I];
    
        % Store parameters in a struct
        params.A = A;
        params.B = B;
    
        % Initialize adaptive parameters if needed
        % params.adaptive_param = ...
    
    end

    function updated_params = update_model_params(params, u2)
        % Implement adaptive parameter update if needed
        % Example:
        % params.adaptive_param = params.adaptive_param + 0.1 * (desired_value - measured_value);
        % ...
    
        % Return the updated parameters
        updated_params = params;
    end
    % Parameters
    Ts = 0.1;  % Sampling time
    N = 10;    % Prediction horizon

    % Update the model parameters if not initialized
    if isempty(model_params)
        model_params = initialize_model_params();
    end

    % State vector (simplified, assuming heading_error is the heading error)
    x = [heading_error; 0];

    % Define cost and constraints for fmincon
    costFunction = @(u) (x + model_params.A * x + model_params.B * u)' * (x + model_params.A * x + model_params.B * u);
    Aeq = [];
    Beq = [];
    Aineq = [];
    Bineq = [];
    lb = -1.5;  % Lower bound on steering input
    ub = 1.5;   % Upper bound on steering input

    % Initial guess
    u0 = 0;

    % Solve optimization problem to get optimal steering input
    options = optimoptions('fmincon', 'Display', 'off', 'Algorithm', 'sqp');
    u_opt = fmincon(costFunction, u0, Aineq, Bineq, Aeq, Beq, lb, ub, [], options);

    % Extract control input (steering angle) from the optimization result
    delta = u_opt;

    % Update model parameters adaptively
    model_params = update_model_params(model_params, u2);
end

== matlab function generic/CarMaker/VehicleControl/CreateBus VhclCtrl1/Stanley steering & speed//Brake controller/Stanley controller with path_planning/Stanley controller with path_planning/Path_Calculation_V02 ==
  data: x_car input; closest_point output; y_car input; path_x input; instantaneous_path output; y_path input
function [closest_point, instantaneous_path] = calculate_path(x_car, y_car, path_x, y_path)
% x_car: x position of the car
% y_car: y position of the car
% path: [2x400] matrix representing the path
path = [path_x;y_path];
%Smoothing the Path
x = path(1,:);
y = path(2,:);
% Define the number of points you want to add for interpolation
num_extra_points = 10000; % Adjust this value as per your requirements
% Compute the total number of points after interpolation
total_points = numel(x) + num_extra_points;
existing_indices = 1:numel(x);
% Create an array of indices for the interpolated points
interpolated_indices = linspace(1, numel(x), total_points);
% Perform spline interpolation on both x and y coordinates
x_interpolated = spline(existing_indices, x, interpolated_indices);
y_interpolated = spline(existing_indices, y, interpolated_indices);

smoothed_path =vertcat(x_interpolated, y_interpolated);
% smoothed_path = smoothed_path_t';


% Calculate the distance between the car and each point on the path
distances = sqrt((smoothed_path(1,:) - x_car).^2 + (smoothed_path(2,:) - y_car).^2);

% Find the index of the closest point on the path
[~, closest_index] = min(distances);

% Get the closest point on the path
closest_point = smoothed_path(:, closest_index);

% Calculate the distance from the closest point to the beginning of the path
distance_to_start = sqrt(sum((smoothed_path(:,closest_index) - smoothed_path(:,1)).^2));

% Calculate the distance from the closest point to the end of the path
distance_to_end = sqrt(sum((smoothed_path(:,closest_index) - smoothed_path(:,end)).^2));

% Determine the number of points to include in the instantaneous path
num_points = min(size(smoothed_path, 2), 20);

% Initialize the instantaneous_path variable using coder.nullcopy
instantaneous_path = coder.nullcopy(zeros(2, num_points));

if distance_to_start < distance_to_end
    % If the closest point is closer to the beginning of the path than the
    % end, include the points starting from the closest point towards the
    % end of the path
    start_index = closest_index;
    end_index = min(size(smoothed_path, 2), closest_index+num_points-1);
else
    % If the closest point is closer to the end of the path than the
    % beginning, include the points starting from the closest point towards
    % the beginning of the path
    start_index = max(1, closest_index-num_points+1);
    end_index = closest_index;
end

%own 
start_index = closest_index;
if start_index > 11139
    end_index = 11159;
    if start_index > 11149
        start_index = 0;
        end_index=20;
    end
else
    end_index = min(size(smoothed_path, 2), closest_index+num_points-1);
end
%own

temp_path = smoothed_path(:, start_index:end_index);
instantaneous_path(:, num_points-size(temp_path, 2)+1:num_points) = temp_path;

end

== matlab function generic/CarMaker/VehicleControl/CreateBus VhclCtrl1/Stanley steering & speed//Brake controller/Stanley controller with path_planning/Stanley controller with path_planning/MATLAB Function1 ==
  data: Pos_X input; Path_Out output; Pos_Y input; Yaw_Angle input; Path_In input
function Path_Out = Abs2RelNew(Pos_X, Pos_Y, Yaw_Angle, Path_In)
%Rotation matrix from absolute to relativ coordination system
R = [cos(Yaw_Angle) sin(Yaw_Angle); -sin(Yaw_Angle) cos(Yaw_Angle)];

Path_X=Path_In(1,:)-Pos_X;      % Shift the points in to the car position
Path_Y=Path_In(2,:)-Pos_Y;      % Shift the points in to the car position
Path=[Path_X;Path_Y];           % Car Point
Path_Out = R*Path;              % Rotate the shifted Points

== matlab function generic/CarMaker/VehicleControl/CreateBus VhclCtrl1/MATLAB Function1 ==
  data: e input; steering output; Cf input; Cr input; v input
function steering = fcn(e,Cf,Cr,v)
%lf = 1.488
%lr = 1.487;
%Cf = 
%Cr =
%m =
% v = 
steering = ((lf+lr)- (lf*Cf-lr*Cr)*m*vx^2)*e...
    /(d_pre*(d_pre+2*L));

== matlab function generic/CarMaker/VehicleControl/CreateBus VhclCtrl1/path_planner_MATLAB/MATLAB Function1 ==
  data: u input; path_x output; path_y output; path_yaw output
function [path_x,path_y,path_yaw] = fcn(u)
path_x = u(1,:);
path_y = u(2,:);
path_yaw = u(3,:);
end

== matlab function generic/CarMaker/VehicleControl/CreateBus VhclCtrl1/path_planner_MATLAB/MATLAB Function ==
  data: path input; e output; yaw input; speed_act input; err_fr_axle output; cross_track_steering output; heading_err output; steering output
function [e, err_fr_axle, cross_track_steering, heading_err, steering]  = conversion(path,yaw,speed_act)
%path = [path_x;path_y];
function distance = calc_distance(pt,v1,v2)
    vect = v1 - v2;
    p_to_vect = pt - v2;
    crossVP = cross(vect,p_to_vect);
    distance = norm(crossVP) / norm(vect) * crossVP(3)/abs(crossVP(3));
end

e = zeros(1);
cross_track_steering = zeros(1);
heading_err = zeros(1);
steering=zeros(1);
err_fr_axle = zeros(1);

k_exp = 1.36;
k_def = 6;
k = k_def + abs(speed_act)^k_exp;
k_ref = 3.1;

% path_index = fix(k_path * speed_act);
% if path_index > 13
%     path_index = 13;
% end
% 
% P_prev = path(:,6 + path_index);
% P_next = path(:,7 + path_index);

fr_axle = [-1.488 0 0];
distances = sqrt((path(1,:) - 1.488).^2 + (path(2,:) - 0).^2);
% Find the index of the closest point on the path
[~,err_fr_axle_ind] = min(distances);
if err_fr_axle_ind == 1
    err_fr_axle_ind = 2;
end
err_fr_axle = calc_distance(fr_axle,[path(1,err_fr_axle_ind - 1) path(2,err_fr_axle_ind - 1) 0],[path(1,err_fr_axle_ind) path(2,err_fr_axle_ind) 0]);

B = [-1.488 + k_ref * (speed_act / 27) 0 0];
distances_err = sqrt((path(1,:) - B(1)).^2 + (path(2,:) - 0).^2);
[~,err_ind] = min(distances_err);
if err_ind < 2
    err_ind = 2;
end
error = calc_distance(B,[path(1,err_ind - 1) path(2,err_ind - 1) 0],[path(1,err_ind) path(2,err_ind) 0]);


P_prev = path(:, err_ind-1);
P_next = path(:, err_ind);

x1 = P_prev(1,1);
y1 = P_prev(2,1);
x2 = P_next(1,1);
y2 = P_next(2,1);

a = (y2 - y1)/-(x2 + x1);
b = 1;
%c = -x1 * (y2 - y1) + y1 * (x2 - x1);


if speed_act ~= 0
    %e = c+b*y1/sqrt((a^2)+(b^2));
    e = error;
    
    cross_track_steering = atan(k * e / speed_act);
    heading_err = atan(-a / b) - yaw;
    %heading_err = 1/(tan(-a/b))-yaw;
    steering = heading_err + cross_track_steering;
end
end

== matlab function generic/CarMaker/VehicleControl/CreateBus VhclCtrl1/path_planner_MATLAB/MATLAB Function2 ==
  data: Pos_X input; Path_Out output; Pos_Y input; Yaw_Angle input; Path_In input
function Path_Out = Abs2RelNew(Pos_X, Pos_Y, Yaw_Angle, Path_In)
%Rotation matrix from absolute to relativ coordination system
R = [cos(Yaw_Angle) sin(Yaw_Angle); -sin(Yaw_Angle) cos(Yaw_Angle)];

Path_X=Path_In(1,:)-Pos_X;      % Shift the points in to the car position
Path_Y=Path_In(2,:)-Pos_Y;      % Shift the points in to the car position
Path=[Path_X;Path_Y];           % Car Point
Path_Out = R*Path;              % Rotate the shifted Points
